simulink library "slController_cl"  (R2020a)
settings: Solver=VariableStepAuto  StartTime=0.0  StopTime=10.0  RelTol=1e-3
undefined symbols (not defined in the file or in its folder): env, FLIGHTCONTROLLER, fltCtrl, initializeBussesFromBlock, thr, vhcl, wnch
libraries: filteredPIDControllerAWGS_ul x4, filteredPIDControllerAW_ul x3, eulAng2RotMat_ul x2, filteredPIDControllerRes_ul x2, simulink x1, ctrlAllocMatrix_cl x1, filteredPIDController_ul x1, alphaBeta_ul x1
settings Model: Creator=jldanie5  LastModifiedBy=andre
settings DataIOCC: ReturnWorkspaceOutputs=off
settings DebuggingCC: ArithmeticOperatorsInVariantConditions=warning
settings SFSimCC: CustomCodeUndefinedFunction=UseInterfaceOnly

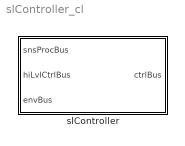
== system slController_cl ==
  slController : Subsystem  LoadFcn=initializeBussesFromBlock(gcb)  InitFcn=initializeBussesFromBlock(gcb)  StartFcn=initializeBussesFromBlock(gcb)  VariantControl=strcmpi(FLIGHTCONTROLLER,'slController')  mask{initPosForInitSStar=vhcl.initPosVecGnd.Value, fluidDensity=env.water.density.Value, LaRCtrl=fltCtrl, aeroStruct=vhcl.struct('OCT.aeroSurf'), LaRThr=thr.tether1, LaRWnch=wnch.winch1}
      mask prompts: initPosForInitSStar "Initial Position"; fluidDensity "Fluid Density"; LaRCtrl "Controller"; aeroStruct "Aerodynamic Structure"; LaRThr "Tether"; LaRWnch "Winch"
      settings: MinAlgLoopOccurrences=on
      mask DialogControl Container3 Prompt: courseFollow Params
      mask DialogControl Container4 Prompt: setpointToOutput Params

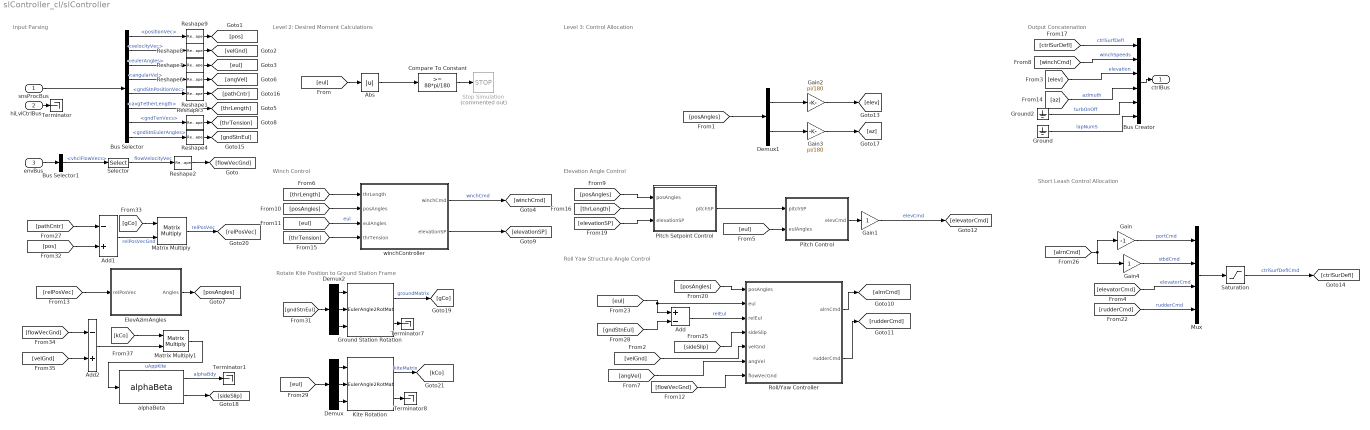
== system slController_cl/slController ==
  note: Rotate Kite Position to Ground Station Frame
  note: Short Leash Control Allocation
  note: Winch Control
  note: Level 3: Control Allocation
  note: Output Concatenation
  note: Level 2: Desired Moment Calculations
  note: Input Parsing
  note: Elevation Angle Control
  note: Roll Yaw Structure Angle Control
  snsProcBus : Inport  OutDataTypeStr=Bus: sensorsProcessingBus
  hiLvlCtrlBus : Inport  Port=2  OutDataTypeStr=Bus: hiLvlCtrlBus
  envBus : Inport  Port=3  OutDataTypeStr=Bus: envBus
  Abs : Abs
  Add : Sum  Inputs=+-
  Add1 : Sum  Inputs=-+
  Add2 : Sum  Inputs=-+
  Bus Creator : BusCreator  Inputs=6  OutDataTypeStr=Bus: fltCtrlBus
      settings: InheritFromInputs=off
  Bus Selector : BusSelector  OutputSignals=positionVec,velocityVec,eulerAngles,angularVel,gndStnPositionVec,avgTetherLength,gndTenVecs,gndStnEulerAngles
  Bus Selector1 : BusSelector  OutputSignals=vhclFlowVecs
  Compare To Constant : simulink/Logic and Bit Operations/Compare To Constant  relop=>=  const=88*pi/180  OutDataTypeStr=boolean
  Demux : Demux  Outputs=3
  Demux1 : Demux  Outputs=2
  Demux2 : Demux  Outputs=3
  ElevAzimAngles : Subsystem
  Gain : Gain  Gain=-1
  Gain1 : Gain
  Gain2 : Gain  Gain=pi/180
  Gain3 : Gain  Gain=pi/180
  Gain4 : Gain
  Ground : Ground
  Ground Station Rotation : eulAng2RotMat_ul/EulerAngle2RotMat  SystemSampleTime=-1  Latency=0  AutoFrameSizeCalculation=off
  Ground2 : Ground
  Kite Rotation : eulAng2RotMat_ul/EulerAngle2RotMat  SystemSampleTime=-1  Latency=0  AutoFrameSizeCalculation=off
  Matrix Multiply : Product  Multiplication=Matrix(*)
  Matrix Multiply1 : Product  Multiplication=Matrix(*)
  Mux : Mux
  Pitch Control : Subsystem
  Pitch Setpoint Control : Subsystem
  Reshape{1..4,6..9} (8 alike) : Reshape  OutputDimensionality=Column vector (2-D)
  Roll/Yaw Controller : Subsystem  Variant=on  VariantControl=Choice
  Saturation : Saturate  UpperLimit=LaRCtrl.controlSigMax.upperLimit.Value  LowerLimit=LaRCtrl.controlSigMax.lowerLimit.Value
  Selector : Selector  NumberOfDimensions=2  InputPortWidth=3  IndexOptions=Select all,Index vector (dialog)  Indices=[1 3],5  OutputSizes=1,1
  Stop Simulation : Stop  Commented=on
  Terminator{,1,7..8} (4 alike) : Terminator
  alphaBeta : alphaBeta_ul/alphaBeta  SystemSampleTime=-1  Latency=0  AutoFrameSizeCalculation=off
  winchController : Subsystem  mask{thrC=LaRThr, ctrlC=LaRCtrl}
      mask prompts: thrC "Tether:"; ctrlC "Controller:"
  ctrlBus : Outport  OutDataTypeStr=Bus: fltCtrlBus  VectorParamsAs1DForOutWhenUnconnected=off
  wires:
  snsProcBus/1 -> Bus Selector/1
  Bus Selector/2 -> Reshape8/1  "<velocityVec>"
  Bus Selector/1 -> Reshape9/1  "<positionVec>"
  Bus Selector/3 -> Reshape7/1  "<eulerAngles>"
  Bus Creator/1 -> ctrlBus/1
  [winchCmd] -> Bus Creator/2  "winchSpeeds"
  [elev] -> Bus Creator/3  "elevation"
  [az] -> Bus Creator/4  "azimuth"
  Bus Selector/4 -> Reshape6/1  "<angularVel>"
  [angVel] -> Roll/Yaw Controller/6(angVel)
  [flowVecGnd] -> Roll/Yaw Controller/7(flowVecGnd)
  [ctrlSurDefl] -> Bus Creator/1  "ctrlSurfDefl"
  Saturation/1 -> [ctrlSurDefl]  "ctrlSurfDeflCmd"
  Reshape2/1 -> [flowVecGnd]
  Reshape6/1 -> [angVel]
  Reshape7/1 -> [eul]
  Reshape8/1 -> [velGnd]
  Reshape9/1 -> [pos]
  Selector/1 -> Reshape2/1  "flowVelocityVec"
  envBus/1 -> Bus Selector1/1
  Bus Selector1/1 -> Selector/1  "<vhclFlowVecs>"
  Reshape1/1 -> [pathCntr]
  Bus Selector/5 -> Reshape1/1  "<gndStnPositionVec>"
  [velGnd] -> Roll/Yaw Controller/5(velGnd)
  hiLvlCtrlBus/1 -> Terminator/1
  [elevatorCmd] -> Mux/3  "elevatorCmd"
  Bus Selector/6 -> [thrLength]  "<avgTetherLength>"
  [thrLength] -> winchController/1(thrLength)
  winchController/1(winchCmd) -> [winchCmd]  "wnchCmd"
  [eul] -> Pitch Control/2(eulAngles)
  Pitch Control/1(elevCmd) -> Gain1/1
  [posAngles] -> Pitch Setpoint Control/1(posAngles)
  Pitch Setpoint Control/1(pitchSP) -> Pitch Control/1(pitchSP)
  Gain1/1 -> [elevatorCmd]  "elevCmd"
  [posAngles] -> winchController/2(posAngles)
  [eul] -> winchController/3(eulAngles)  "eul"
  Ground2/1 -> Bus Creator/5  "turbOnOff"
  [relPosVec] -> ElevAzimAngles/1(relPosVec)
  ElevAzimAngles/1(Angles) -> [posAngles]
  Bus Selector/7 -> Reshape3/1  "<gndTenVecs>"
  [thrTension] -> winchController/4(thrTension)
  Reshape3/1 -> [thrTension]
  [thrLength] -> ?
  winchController/2(elevationSP) -> [elevationSP]
  [elevationSP] -> Pitch Setpoint Control/2(elevationSP)
  [rudderCmd] -> Mux/4  "rudderCmd"
  Gain/1 -> Mux/1  "portCmd"
  [alrnCmd] -> Gain4/1, Gain/1
  Mux/1 -> Saturation/1
  Bus Selector/8 -> Reshape4/1  "<gndStnEulerAngles>"
  Reshape4/1 -> [gndStnEul]
  [eul] -> Demux/1
  Demux/1 -> Kite Rotation/1
  Demux/2 -> Kite Rotation/2
  Demux/3 -> Kite Rotation/3
  [gndStnEul] -> Demux2/1
  Demux2/1 -> Ground Station Rotation/1
  Demux2/2 -> Ground Station Rotation/2
  Demux2/3 -> Ground Station Rotation/3
  Kite Rotation/1 -> [kCo]  "kiteMatrix"
  Ground Station Rotation/2 -> Terminator7/1
  Ground Station Rotation/1 -> [gCo]  "groundMatrix"
  Kite Rotation/2 -> Terminator8/1
  Add1/1 -> Matrix Multiply/2  "relPosVecGnd"
  [pathCntr] -> Add1/1
  [pos] -> Add1/2
  [gCo] -> Matrix Multiply/1
  Matrix Multiply/1 -> [relPosVec]  "relPosVec"
  [velGnd] -> Add2/2
  [flowVecGnd] -> Add2/1
  alphaBeta/2 -> [sideSlip]
  Add2/1 -> Matrix Multiply1/2
  [kCo] -> Matrix Multiply1/1
  Matrix Multiply1/1 -> alphaBeta/1  "uAppKite"
  [gndStnEul] -> Add/2
  [eul] -> Add/1, Roll/Yaw Controller/2(eul)
  [posAngles] -> Roll/Yaw Controller/1(posAngles)
  Roll/Yaw Controller/1(alrnCmd) -> [alrnCmd]
  Roll/Yaw Controller/2(rudderCmd) -> [rudderCmd]
  [sideSlip] -> Roll/Yaw Controller/4(sideSlip)
  Add/1 -> Roll/Yaw Controller/3(relEul)  "relEul"
  [eul] -> Abs/1
  Abs/1 -> Compare To Constant/1
  Compare To Constant/1 -> Stop Simulation/1
  [posAngles] -> Demux1/1
  Demux1/1 -> Gain2/1
  Demux1/2 -> Gain3/1
  Gain2/1 -> [elev]
  Gain3/1 -> [az]
  Gain4/1 -> Mux/2  "stbdCmd"
  alphaBeta/1 -> Terminator1/1  "alphaBdy"
  Ground/1 -> Bus Creator/6  "lapNumS"

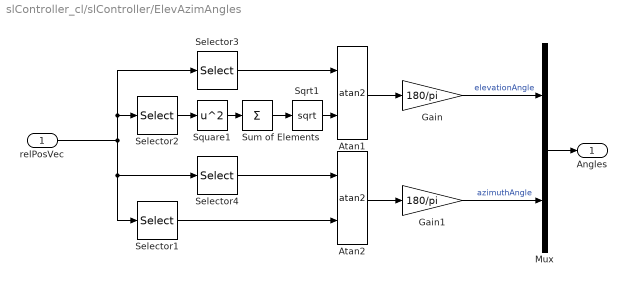
== system slController_cl/slController/ElevAzimAngles ==
  relPosVec : Inport
  Atan1 : Trigonometry  Operator=atan2
  Atan2 : Trigonometry  Operator=atan2
  Gain : Gain  Gain=180/pi
  Gain1 : Gain  Gain=180/pi
  Mux : Mux  Inputs=2
  Selector1 : Selector  InputPortWidth=3  IndexOptions=Index vector (dialog)  Indices=1  OutputSizes=1
  Selector2 : Selector  InputPortWidth=3  IndexOptions=Index vector (dialog)  Indices=[1 2]  OutputSizes=1
  Selector3 : Selector  InputPortWidth=3  IndexOptions=Index vector (dialog)  Indices=3  OutputSizes=1
  Selector4 : Selector  InputPortWidth=3  IndexOptions=Index vector (dialog)  Indices=2  OutputSizes=1
  Sqrt1 : Sqrt  SaturateOnIntegerOverflow=on
  Square1 : Math  Operator=square  SignedPower=on  SaturateOnIntegerOverflow=on
  Sum of Elements : Sum  Inputs=+
  Angles : Outport
  wires:
  Sqrt1/1 -> Atan1/2
  Square1/1 -> Sum of Elements/1
  Selector3/1 -> Atan1/1
  Sum of Elements/1 -> Sqrt1/1
  Atan1/1 -> Gain/1
  Selector2/1 -> Square1/1
  Selector4/1 -> Atan2/1
  relPosVec/1 -> Selector3/1, Selector2/1, Selector4/1, Selector1/1
  Atan2/1 -> Gain1/1
  Selector1/1 -> Atan2/2
  Gain/1 -> Mux/1  "elevationAngle"
  Gain1/1 -> Mux/2  "azimuthAngle"
  Mux/1 -> Angles/1

== system slController_cl/slController/Pitch Control ==
  pitchSP : Inport
  eulAngles : Inport  Port=2
  Add1 : Sum  Inputs=-+
  Gain2 : Gain  Gain=pi/180
  Selector2 : Selector  InputPortWidth=3  IndexOptions=Index vector (dialog)  Indices=2  OutputSizes=1
  filteredPIDControllerAW : filteredPIDControllerAW_ul/filteredPIDControllerAW  kp=LaRCtrl.elevCmd.kp.Value  ki=LaRCtrl.elevCmd.ki.Value  kd=LaRCtrl.elevCmd.kd.Value  tau=LaRCtrl.elevCmd.tau.Value  cmax=LaRCtrl.controlSigMax.upperLimit.Value  cmin=LaRCtrl.controlSigMax.lowerLimit.Value
  elevCmd : Outport
  wires:
  Selector2/1 -> Add1/2  "pitch"
  filteredPIDControllerAW/1 -> elevCmd/1  "elevCmd"
  pitchSP/1 -> Gain2/1
  eulAngles/1 -> Selector2/1
  Gain2/1 -> Add1/1
  Add1/1 -> filteredPIDControllerAW/1  "err"

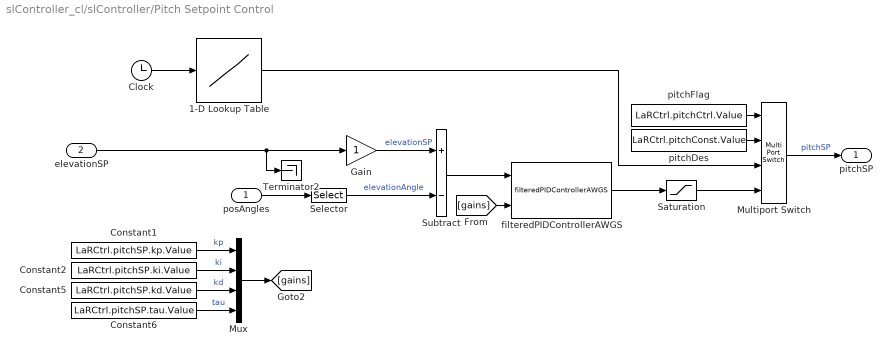
== system slController_cl/slController/Pitch Setpoint Control ==
  posAngles : Inport
  elevationSP : Inport  Port=2
  1-D Lookup Table : Lookup_n-D  NumberOfTableDimensions=1  BreakpointsForDimension1=LaRCtrl.pitchTime.Value  Table=LaRCtrl.pitchLookup.Value  InterpMethod=Flat  InternalRulePriority=Speed  RndMeth=Simplest  InputSameDT=on
  Clock : Clock
  Constant1 : Constant  Value=LaRCtrl.pitchSP.kp.Value
  Constant2 : Constant  Value=LaRCtrl.pitchSP.ki.Value
  Constant5 : Constant  Value=LaRCtrl.pitchSP.kd.Value
  Constant6 : Constant  Value=LaRCtrl.pitchSP.tau.Value
  Gain : Gain
  Multiport Switch : MultiPortSwitch  DataPortOrder=Specify indices  Inputs=2  DataPortIndices={0,1,2}
  Mux : Mux
  Saturation : Saturate  UpperLimit=LaRCtrl.pitchAngleMax.upperLimit.Value  LowerLimit=LaRCtrl.pitchAngleMax.lowerLimit.Value
  Selector : Selector  InputPortWidth=2  IndexOptions=Index vector (dialog)  Indices=1  OutputSizes=1
  Subtract : Sum  Inputs=+-
  Terminator2 : Terminator
  filteredPIDControllerAWGS : filteredPIDControllerAWGS_ul/filteredPIDControllerAWGS  cmax=LaRCtrl.pitchAngleMax.upperLimit.Value  cmin=LaRCtrl.pitchAngleMax.lowerLimit.Value
  pitchDes : Constant  Value=LaRCtrl.pitchConst.Value
  pitchFlag : Constant  Value=LaRCtrl.pitchCtrl.Value
  pitchSP : Outport
  wires:
  pitchFlag/1 -> Multiport Switch/1
  Multiport Switch/1 -> pitchSP/1  "pitchSP"
  pitchDes/1 -> Multiport Switch/2
  posAngles/1 -> Selector/1
  Clock/1 -> 1-D Lookup Table/1
  Selector/1 -> Subtract/2  "elevationAngle"
  Gain/1 -> Subtract/1  "elevationSP"
  1-D Lookup Table/1 -> Multiport Switch/3
  elevationSP/1 -> Gain/1, Terminator2/1
  Subtract/1 -> filteredPIDControllerAWGS/1
  Constant1/1 -> Mux/1  "kp"
  Constant2/1 -> Mux/2  "ki"
  Constant5/1 -> Mux/3  "kd"
  Constant6/1 -> Mux/4  "tau"
  [gains] -> filteredPIDControllerAWGS/2
  Mux/1 -> [gains]
  filteredPIDControllerAWGS/1 -> Saturation/1
  Saturation/1 -> Multiport Switch/4

== system slController_cl/slController/Roll//Yaw Controller ==
  posAngles : Inport
  eul : Inport  Port=2
  relEul : Inport  Port=3
  sideSlip : Inport  Port=4
  velGnd : Inport  Port=5
  angVel : Inport  Port=6
  flowVecGnd : Inport  Port=7
  NDICtrl : Subsystem  VariantControl=strcmpi(fltCtrl.towCtrlStrat.Value,'NDICtrl')
  rollAzYawSide : Subsystem  VariantControl=strcmpi(fltCtrl.towCtrlStrat.Value,'rollAzYawSide')
  yawAz : Subsystem  VariantControl=strcmpi(fltCtrl.towCtrlStrat.Value,'yawAz')
  alrnCmd : Outport
  rudderCmd : Outport  Port=2

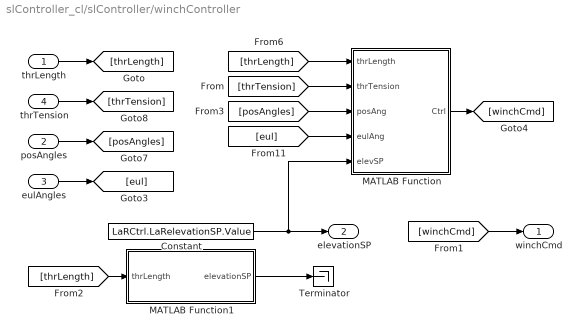
== system slController_cl/slController/winchController ==
  thrLength : Inport
  posAngles : Inport  Port=2
  eulAngles : Inport  Port=3
  thrTension : Inport  Port=4
  Constant : Constant  Value=LaRCtrl.LaRelevationSP.Value
  MATLAB Function : MATLAB Function  TreatAsAtomicUnit=on  mask{leash=LaRCtrl.shortLeashLength.Value, spd=LaRCtrl.nomSpoolSpeed.Value, coneWidth=LaRCtrl.LaRelevationSPErr.Value}
      mask prompts: leash "Short Leash Length [m]"; spd "Nominal Spool Speed [m/s]"; coneWidth "Elevation Angle Error Threshold"
  MATLAB Function1 : MATLAB Function  TreatAsAtomicUnit=on  mask{elevSP1=LaRCtrl.LaRelevationSP.Value, elevSP2=50}
      mask prompts: elevSP1 "Nominal Elevation Setpoint [deg]"; elevSP2 "Final Elevation Setpoint [deg]"
  Terminator : Terminator
  winchCmd : Outport
  elevationSP : Outport  Port=2
  wires:
  thrLength/1 -> [thrLength]
  posAngles/1 -> [posAngles]
  [winchCmd] -> winchCmd/1
  eulAngles/1 -> [eul]
  [eul] -> MATLAB Function/4(eulAng)
  [posAngles] -> MATLAB Function/3(posAng)
  [thrLength] -> MATLAB Function/1(thrLength)
  thrTension/1 -> [thrTension]
  [thrTension] -> MATLAB Function/2(thrTension)
  MATLAB Function/1(Ctrl) -> [winchCmd]
  [thrLength] -> MATLAB Function1/1(thrLength)
  Constant/1 -> MATLAB Function/5(elevSP), elevationSP/1
  MATLAB Function1/1(elevationSP) -> Terminator/1

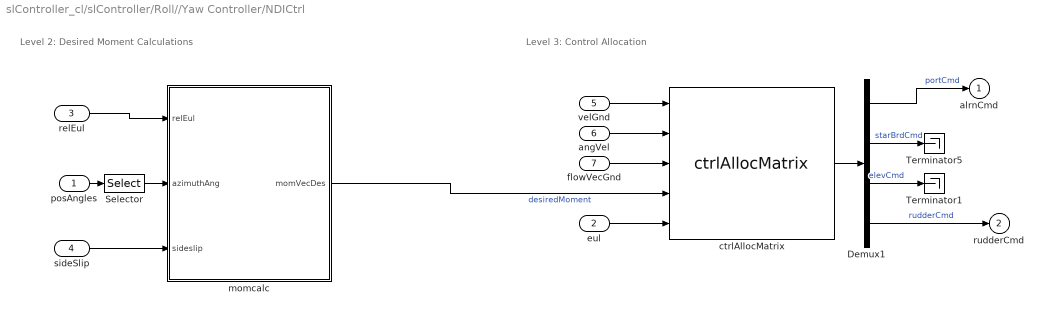
== system slController_cl/slController/Roll//Yaw Controller/NDICtrl ==
  note: Level 2: Desired Moment Calculations
  note: Level 3: Control Allocation
  posAngles : Inport
  eul : Inport  Port=2
  relEul : Inport  Port=3
  sideSlip : Inport  Port=4
  velGnd : Inport  Port=5
  angVel : Inport  Port=6
  flowVecGnd : Inport  Port=7
  Demux1 : Demux
  Selector : Selector  InputPortWidth=3  IndexOptions=Index vector (dialog)  Indices=2  OutputSizes=1
  Terminator1 : Terminator
  Terminator5 : Terminator
  ctrlAllocMatrix : ctrlAllocMatrix_cl/ctrlAllocMatrix  aeroStruct=aeroStruct  fluidDensity=fluidDensity
  momcalc : Subsystem
  alrnCmd : Outport
  rudderCmd : Outport  Port=2
  wires:
  Demux1/2 -> Terminator5/1  "starBrdCmd"
  Demux1/4 -> rudderCmd/1  "rudderCmd"
  relEul/1 -> momcalc/1(relEul)
  eul/1 -> ctrlAllocMatrix/5
  Demux1/1 -> alrnCmd/1  "portCmd"
  Demux1/3 -> Terminator1/1  "elevCmd"
  momcalc/1(momVecDes) -> ctrlAllocMatrix/4  "desiredMoment"
  flowVecGnd/1 -> ctrlAllocMatrix/3
  angVel/1 -> ctrlAllocMatrix/2
  ctrlAllocMatrix/1 -> Demux1/1
  velGnd/1 -> ctrlAllocMatrix/1
  posAngles/1 -> Selector/1
  Selector/1 -> momcalc/2(azimuthAng)
  sideSlip/1 -> momcalc/3(sideslip)

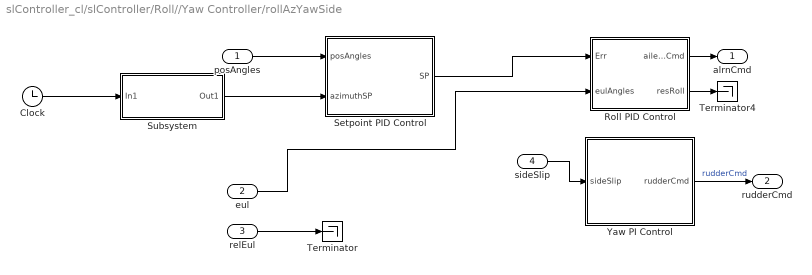
== system slController_cl/slController/Roll//Yaw Controller/rollAzYawSide ==
  posAngles : Inport
  eul : Inport  Port=2
  relEul : Inport  Port=3
  sideSlip : Inport  Port=4
  Clock : Clock
  Roll PID Control : Subsystem
  Setpoint PID Control : Subsystem
  Subsystem : Subsystem
  Terminator : Terminator
  Terminator4 : Terminator
  Yaw PI Control : Subsystem
  alrnCmd : Outport
  rudderCmd : Outport  Port=2
  wires:
  Subsystem/1(Out1) -> Setpoint PID Control/2(azimuthSP)
  Yaw PI Control/1(rudderCmd) -> rudderCmd/1  "rudderCmd"
  Roll PID Control/1(aileronCmd) -> alrnCmd/1
  eul/1 -> Roll PID Control/2(eulAngles)
  relEul/1 -> Terminator/1
  Roll PID Control/2(resRoll) -> Terminator4/1
  Setpoint PID Control/1(SP) -> Roll PID Control/1(Err)
  sideSlip/1 -> Yaw PI Control/1(sideSlip)
  posAngles/1 -> Setpoint PID Control/1(posAngles)
  Clock/1 -> Subsystem/1(In1)

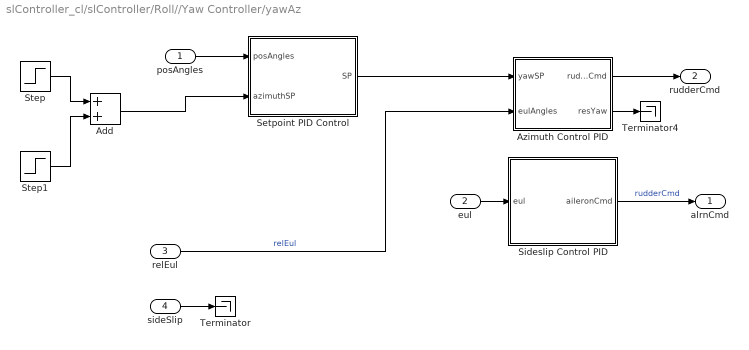
== system slController_cl/slController/Roll//Yaw Controller/yawAz ==
  posAngles : Inport
  eul : Inport  Port=2
  relEul : Inport  Port=3
  sideSlip : Inport  Port=4
  Add : Sum
  Azimuth Control PID : Subsystem
  Setpoint PID Control : Subsystem
  Sideslip Control PID : Subsystem
  Step : Step  Time=300  After=10  SampleTime=0
  Step1 : Step  Time=300  After=-10  SampleTime=0
  Terminator : Terminator
  Terminator4 : Terminator
  alrnCmd : Outport
  rudderCmd : Outport  Port=2
  wires:
  posAngles/1 -> Setpoint PID Control/1(posAngles)
  Setpoint PID Control/1(SP) -> Azimuth Control PID/1(yawSP)
  Azimuth Control PID/2(resYaw) -> Terminator4/1
  relEul/1 -> Azimuth Control PID/2(eulAngles)  "relEul"
  Sideslip Control PID/1(aileronCmd) -> alrnCmd/1  "rudderCmd"
  sideSlip/1 -> Terminator/1
  eul/1 -> Sideslip Control PID/1(eul)
  Step1/1 -> Add/2
  Step/1 -> Add/1
  Add/1 -> Setpoint PID Control/2(azimuthSP)
  Azimuth Control PID/1(rudderCmd) -> rudderCmd/1

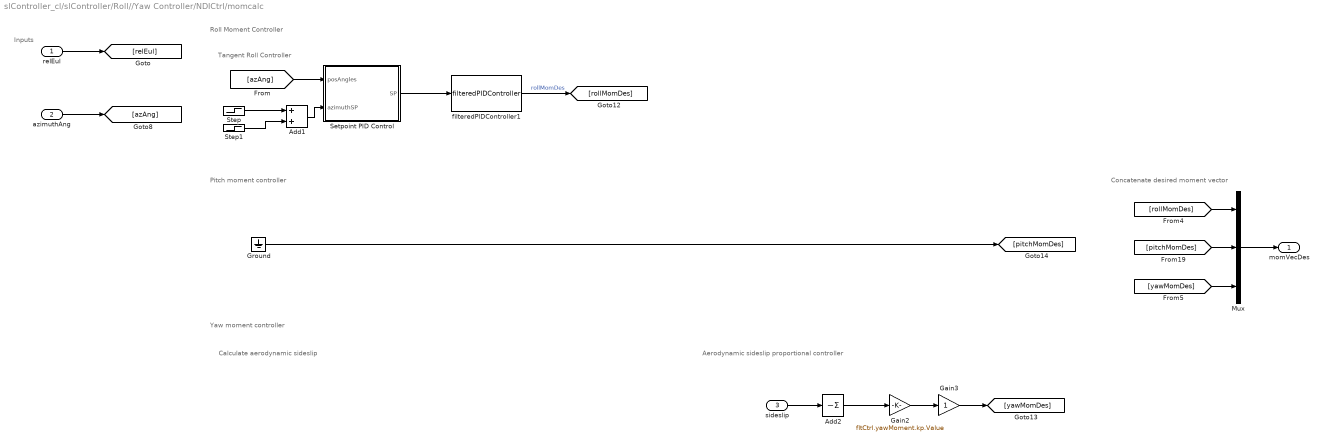
== system slController_cl/slController/Roll//Yaw Controller/NDICtrl/momcalc ==
  note: Roll Moment Controller
  note: Pitch moment controller
  note: Yaw moment controller
  note: Calculate aerodynamic sideslip
  note: Aerodynamic sideslip proportional controller
  note: Concatenate desired moment vector
  note: Tangent Roll Controller
  note: Inputs
  relEul : Inport
  azimuthAng : Inport  Port=2
  sideslip : Inport  Port=3
  Add1 : Sum
  Add2 : Sum  Inputs=-
  Gain2 : Gain  Gain=fltCtrl.yawMoment.kp.Value
  Gain3 : Gain
  Ground : Ground
  Mux : Mux  Inputs=3
  Setpoint PID Control : Subsystem
  Step : Step  Time=300  After=10  SampleTime=0
  Step1 : Step  Time=300  After=-10  SampleTime=0
  filteredPIDController1 : filteredPIDController_ul/filteredPIDController  kp=LaRCtrl.rollMoment.kp.Value  ki=LaRCtrl.rollMoment.ki.Value  kd=LaRCtrl.rollMoment.kd.Value  Value=LaRCtrl.rollMoment.tau.Value  externalReset=none
  momVecDes : Outport  VectorParamsAs1DForOutWhenUnconnected=off
  wires:
  azimuthAng/1 -> [azAng]
  Ground/1 -> [pitchMomDes]
  relEul/1 -> [relEul]
  filteredPIDController1/1 -> [rollMomDes]  "rollMomDes"
  Gain2/1 -> Gain3/1
  Setpoint PID Control/1(SP) -> filteredPIDController1/1
  Mux/1 -> momVecDes/1
  Gain3/1 -> [yawMomDes]
  [pitchMomDes] -> Mux/2
  [rollMomDes] -> Mux/1
  [yawMomDes] -> Mux/3
  Step/1 -> Add1/1
  Step1/1 -> Add1/2
  [azAng] -> Setpoint PID Control/1(posAngles)
  Add1/1 -> Setpoint PID Control/2(azimuthSP)
  sideslip/1 -> Add2/1
  Add2/1 -> Gain2/1

== system slController_cl/slController/Roll//Yaw Controller/rollAzYawSide/Roll PID Control ==
  Err : Inport
  eulAngles : Inport  Port=2
  Add1 : Sum  Inputs=+-
  Gain : Gain
  Gain1 : Gain  Gain=-1
  Gain3 : Gain  Gain=-1
  Selector2 : Selector  InputPortWidth=3  IndexOptions=Index vector (dialog)  Indices=1  OutputSizes=1
  Terminator : Terminator
  filteredPIDControllerRes : filteredPIDControllerRes_ul/filteredPIDControllerRes  kp=LaRCtrl.alrnCmd.kp.Value  ki=LaRCtrl.alrnCmd.ki.Value  kd=LaRCtrl.alrnCmd.kd.Value  Value=LaRCtrl.alrnCmd.tau.Value  UpperLimit=LaRCtrl.controlSigMax.upperLimit.Value  LowerLimit=LaRCtrl.controlSigMax.lowerLimit.Value  externalReset=none
  aileronCmd : Outport
  resRoll : Outport  Port=2
  wires:
  filteredPIDControllerRes/1 -> Gain1/1  "aileronCMD"
  eulAngles/1 -> Selector2/1
  Selector2/1 -> Gain3/1  "roll"
  Add1/1 -> filteredPIDControllerRes/1  "rollErr"
  Err/1 -> Gain/1
  filteredPIDControllerRes/3 -> Terminator/1
  Gain1/1 -> aileronCmd/1
  filteredPIDControllerRes/2 -> resRoll/1
  Gain3/1 -> Add1/2  "roll"
  Gain/1 -> Add1/1  "rollSP"

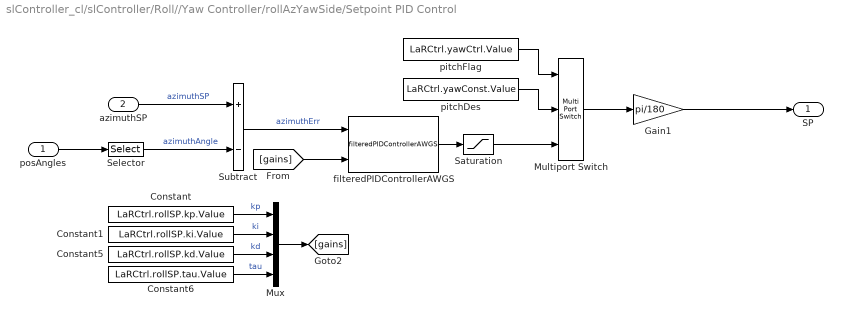
== system slController_cl/slController/Roll//Yaw Controller/rollAzYawSide/Setpoint PID Control ==
  posAngles : Inport
  azimuthSP : Inport  Port=2
  Constant : Constant  Value=LaRCtrl.rollSP.kp.Value
  Constant1 : Constant  Value=LaRCtrl.rollSP.ki.Value
  Constant5 : Constant  Value=LaRCtrl.rollSP.kd.Value
  Constant6 : Constant  Value=LaRCtrl.rollSP.tau.Value
  Gain1 : Gain  Gain=pi/180
  Multiport Switch : MultiPortSwitch  DataPortOrder=Specify indices  Inputs=2  DataPortIndices={0,1}
  Mux : Mux
  Saturation : Saturate  UpperLimit=LaRCtrl.pitchAngleMax.upperLimit.Value  LowerLimit=LaRCtrl.pitchAngleMax.lowerLimit.Value
  Selector : Selector  InputPortWidth=2  IndexOptions=Index vector (dialog)  Indices=2  OutputSizes=1
  Subtract : Sum  Inputs=+-
  filteredPIDControllerAWGS : filteredPIDControllerAWGS_ul/filteredPIDControllerAWGS  cmax=LaRCtrl.pitchAngleMax.upperLimit.Value  cmin=LaRCtrl.pitchAngleMax.lowerLimit.Value
  pitchDes : Constant  Value=LaRCtrl.yawConst.Value
  pitchFlag : Constant  Value=LaRCtrl.yawCtrl.Value
  SP : Outport
  wires:
  pitchFlag/1 -> Multiport Switch/1
  Multiport Switch/1 -> Gain1/1
  pitchDes/1 -> Multiport Switch/2
  posAngles/1 -> Selector/1
  Selector/1 -> Subtract/2  "azimuthAngle"
  azimuthSP/1 -> Subtract/1  "azimuthSP"
  Subtract/1 -> filteredPIDControllerAWGS/1  "azimuthErr"
  Constant/1 -> Mux/1  "kp"
  Constant1/1 -> Mux/2  "ki"
  Constant5/1 -> Mux/3  "kd"
  Constant6/1 -> Mux/4  "tau"
  Mux/1 -> [gains]
  filteredPIDControllerAWGS/1 -> Saturation/1
  Saturation/1 -> Multiport Switch/3
  [gains] -> filteredPIDControllerAWGS/2
  Gain1/1 -> SP/1

== system slController_cl/slController/Roll//Yaw Controller/rollAzYawSide/Subsystem ==
  In1 : Inport
  1-D Lookup Table : Lookup_n-D  NumberOfTableDimensions=1  BreakpointsForDimension1=[0 100 100.1 100.2]  Table=[0 0 0 0]  InternalRulePriority=Speed  RndMeth=Simplest  InputSameDT=on
  Out1 : Outport
  wires:
  In1/1 -> 1-D Lookup Table/1
  1-D Lookup Table/1 -> Out1/1

== system slController_cl/slController/Roll//Yaw Controller/rollAzYawSide/Yaw PI Control ==
  sideSlip : Inport
  Gain : Gain  Gain=-1
  Gain3 : Gain  Gain=-pi/180
  filteredPIDControllerAW : filteredPIDControllerAW_ul/filteredPIDControllerAW  kp=LaRCtrl.rudderCmd.kp.Value  ki=LaRCtrl.rudderCmd.ki.Value  kd=LaRCtrl.rudderCmd.kd.Value  tau=LaRCtrl.rudderCmd.tau.Value  cmax=LaRCtrl.controlSigMax.upperLimit.Value  cmin=LaRCtrl.controlSigMax.lowerLimit.Value
  rudderCmd : Outport
  wires:
  Gain3/1 -> filteredPIDControllerAW/1  "yawErr"
  sideSlip/1 -> Gain3/1  "yawSP"
  Gain/1 -> rudderCmd/1
  filteredPIDControllerAW/1 -> Gain/1  "rudderCmd"

== system slController_cl/slController/Roll//Yaw Controller/yawAz/Azimuth Control PID ==
  yawSP : Inport
  eulAngles : Inport  Port=2
  Add1 : Sum  Inputs=+-
  Gain1 : Gain  Gain=-1
  Selector2 : Selector  InputPortWidth=3  IndexOptions=Index vector (dialog)  Indices=3  OutputSizes=1
  Terminator : Terminator
  filteredPIDControllerRes : filteredPIDControllerRes_ul/filteredPIDControllerRes  kp=LaRCtrl.rudderCmd.kp.Value  ki=LaRCtrl.rudderCmd.ki.Value  kd=LaRCtrl.rudderCmd.kd.Value  Value=LaRCtrl.rudderCmd.tau.Value  UpperLimit=LaRCtrl.controlSigMax.upperLimit.Value  LowerLimit=LaRCtrl.controlSigMax.lowerLimit.Value  externalReset=none
  rudderCmd : Outport
  resYaw : Outport  Port=2
  wires:
  yawSP/1 -> Add1/1  "yawSP"
  filteredPIDControllerRes/2 -> resYaw/1
  Gain1/1 -> rudderCmd/1
  filteredPIDControllerRes/3 -> Terminator/1
  Add1/1 -> filteredPIDControllerRes/1  "yawErr"
  Selector2/1 -> Add1/2  "yaw"
  eulAngles/1 -> Selector2/1
  filteredPIDControllerRes/1 -> Gain1/1  "rudder"

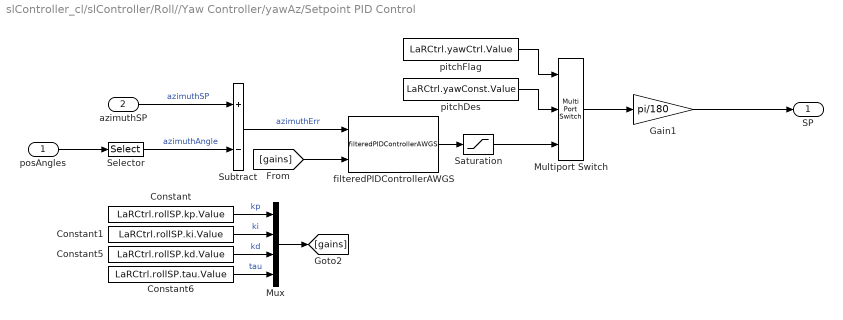
== system slController_cl/slController/Roll//Yaw Controller/yawAz/Setpoint PID Control ==
  posAngles : Inport
  azimuthSP : Inport  Port=2
  Constant : Constant  Value=LaRCtrl.rollSP.kp.Value
  Constant1 : Constant  Value=LaRCtrl.rollSP.ki.Value
  Constant5 : Constant  Value=LaRCtrl.rollSP.kd.Value
  Constant6 : Constant  Value=LaRCtrl.rollSP.tau.Value
  Gain1 : Gain  Gain=pi/180
  Multiport Switch : MultiPortSwitch  DataPortOrder=Specify indices  Inputs=2  DataPortIndices={0,1}
  Mux : Mux
  Saturation : Saturate  UpperLimit=LaRCtrl.pitchAngleMax.upperLimit.Value  LowerLimit=LaRCtrl.pitchAngleMax.lowerLimit.Value
  Selector : Selector  InputPortWidth=2  IndexOptions=Index vector (dialog)  Indices=2  OutputSizes=1
  Subtract : Sum  Inputs=+-
  filteredPIDControllerAWGS : filteredPIDControllerAWGS_ul/filteredPIDControllerAWGS  cmax=LaRCtrl.pitchAngleMax.upperLimit.Value  cmin=LaRCtrl.pitchAngleMax.lowerLimit.Value
  pitchDes : Constant  Value=LaRCtrl.yawConst.Value
  pitchFlag : Constant  Value=LaRCtrl.yawCtrl.Value
  SP : Outport
  wires:
  Gain1/1 -> SP/1
  [gains] -> filteredPIDControllerAWGS/2
  Saturation/1 -> Multiport Switch/3
  filteredPIDControllerAWGS/1 -> Saturation/1
  Mux/1 -> [gains]
  Constant6/1 -> Mux/4  "tau"
  Constant5/1 -> Mux/3  "kd"
  Constant1/1 -> Mux/2  "ki"
  Constant/1 -> Mux/1  "kp"
  Subtract/1 -> filteredPIDControllerAWGS/1  "azimuthErr"
  azimuthSP/1 -> Subtract/1  "azimuthSP"
  Selector/1 -> Subtract/2  "azimuthAngle"
  posAngles/1 -> Selector/1
  pitchDes/1 -> Multiport Switch/2
  Multiport Switch/1 -> Gain1/1
  pitchFlag/1 -> Multiport Switch/1

== system slController_cl/slController/Roll//Yaw Controller/yawAz/Sideslip Control PID ==
  eul : Inport
  Gain : Gain
  Gain1 : Gain  Gain=-1
  Selector : Selector  InputPortWidth=3  IndexOptions=Index vector (dialog)  Indices=1  OutputSizes=1
  filteredPIDControllerAW : filteredPIDControllerAW_ul/filteredPIDControllerAW  kp=LaRCtrl.alrnCmd.kp.Value  ki=LaRCtrl.alrnCmd.ki.Value  kd=LaRCtrl.alrnCmd.kd.Value  tau=LaRCtrl.alrnCmd.tau.Value  cmax=LaRCtrl.controlSigMax.upperLimit.Value  cmin=LaRCtrl.controlSigMax.lowerLimit.Value
  aileronCmd : Outport
  wires:
  Selector/1 -> Gain1/1
  filteredPIDControllerAW/1 -> Gain/1  "aileronCmd"
  Gain/1 -> aileronCmd/1
  eul/1 -> Selector/1  "SP"
  Gain1/1 -> filteredPIDControllerAW/1

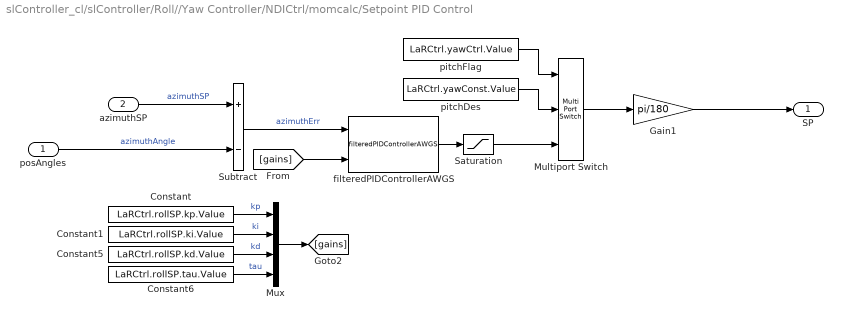
== system slController_cl/slController/Roll//Yaw Controller/NDICtrl/momcalc/Setpoint PID Control ==
  posAngles : Inport
  azimuthSP : Inport  Port=2
  Constant : Constant  Value=LaRCtrl.rollSP.kp.Value
  Constant1 : Constant  Value=LaRCtrl.rollSP.ki.Value
  Constant5 : Constant  Value=LaRCtrl.rollSP.kd.Value
  Constant6 : Constant  Value=LaRCtrl.rollSP.tau.Value
  Gain1 : Gain  Gain=pi/180
  Multiport Switch : MultiPortSwitch  DataPortOrder=Specify indices  Inputs=2  DataPortIndices={0,1}
  Mux : Mux
  Saturation : Saturate  UpperLimit=LaRCtrl.pitchAngleMax.upperLimit.Value  LowerLimit=LaRCtrl.pitchAngleMax.lowerLimit.Value
  Subtract : Sum  Inputs=+-
  filteredPIDControllerAWGS : filteredPIDControllerAWGS_ul/filteredPIDControllerAWGS  cmax=LaRCtrl.pitchAngleMax.upperLimit.Value  cmin=LaRCtrl.pitchAngleMax.lowerLimit.Value
  pitchDes : Constant  Value=LaRCtrl.yawConst.Value
  pitchFlag : Constant  Value=LaRCtrl.yawCtrl.Value
  SP : Outport
  wires:
  Gain1/1 -> SP/1
  [gains] -> filteredPIDControllerAWGS/2
  Saturation/1 -> Multiport Switch/3
  filteredPIDControllerAWGS/1 -> Saturation/1
  Mux/1 -> [gains]
  Constant6/1 -> Mux/4  "tau"
  Constant5/1 -> Mux/3  "kd"
  Constant1/1 -> Mux/2  "ki"
  Constant/1 -> Mux/1  "kp"
  Subtract/1 -> filteredPIDControllerAWGS/1  "azimuthErr"
  azimuthSP/1 -> Subtract/1  "azimuthSP"
  posAngles/1 -> Subtract/2  "azimuthAngle"
  pitchDes/1 -> Multiport Switch/2
  Multiport Switch/1 -> Gain1/1
  pitchFlag/1 -> Multiport Switch/1

== matlab function slController_cl/slController/winchController/MATLAB Function1 ==
  data: thrLength input; elevationSP output; elevSP1 parameter; elevSP2 parameter
function elevationSP = fcn(thrLength,elevSP1, elevSP2)

if thrLength > 95
    elevationSP = elevSP1;
else
    elevationSP = elevSP2;
end

== matlab function slController_cl/slController/winchController/MATLAB Function ==
  data: thrLength input; thrTension input; posAng input; Ctrl output; eulAng input; coneWidth parameter; leash parameter; spd parameter; elevSP input
function Ctrl  = fcn(thrLength, thrTension, posAng, eulAng, coneWidth, leash, spd, elevSP)

roll = eulAng(1)*180/pi;                                %   deg - Roll angle 
% pitch = eulAng(2)*180/pi;                               %   deg - Pitch angle 
% yaw = eulAng(3)*180/pi;                                 %   deg - Yaw angle 

elevationAngle = posAng(1);                             %   deg - Elevation angle 
elevationError = abs(elevSP-elevationAngle);            %   deg - Elevation angle error 
% if thrLength < 100
%     spd = spd;
% end
nomWidth = coneWidth/2;                                 %   deg - Width of elevation cone where nominal speed is allowed
x = [nomWidth coneWidth];
y = [-spd 0];
m = (y(2)-y(1))/(x(2)-x(1));

thrErr = thrLength-leash;                               %   m - Tether length error 

if abs(roll) > 2.5
    Ctrl = 0;
elseif elevationError <= coneWidth
    if thrErr > 1
        Ctrl = max(min(m*(elevationError-x(1))+y(1),0),-spd);
    else
        Ctrl = 0;
    end
else
    Ctrl = 0;
end
